simulink model "simulinkQ1b (1)"  (R2022a)
settings: Solver=VariableStepAuto  StartTime=0.0  StopTime=10.0  RelTol=1e-3
settings Model: Creator=ABHIJIT NIT  LastModifiedBy=heera
settings DebuggingCC: UnconnectedInputMsg=warning  UnconnectedOutputMsg=warning  UnconnectedLineMsg=warning
settings RTWCC: DLArmComputeVersion=19.05

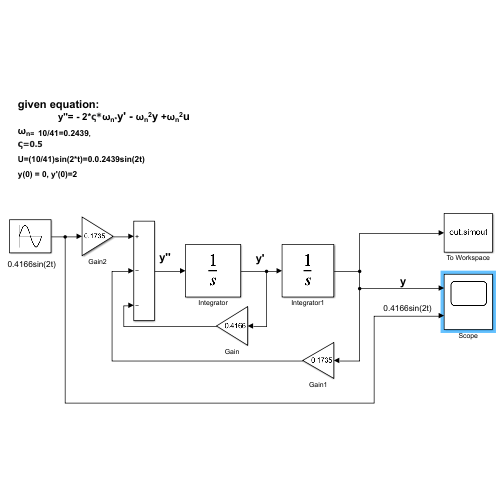
[thumbnail: Simulink's stored preview of the top-level diagram]
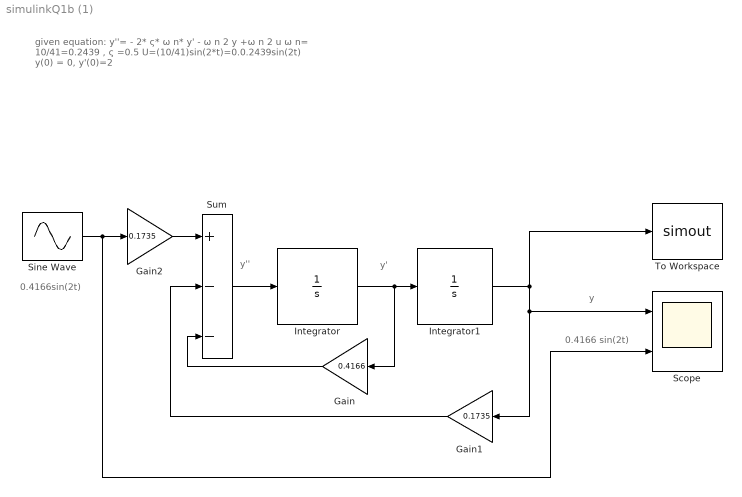
== system simulinkQ1b (1) ==
  note: 0.4166 sin(2t)
  note: 0.4166sin(2t)
  note: y''
  note: given equation:
      | y''= - 2* ς* ω n* y' - ω n 2 y +ω n 2 u
      | ω n= 10/41=0.2439 ,
      | ς =0.5
      | U=(10/41)sin(2*t)=0.0.2439sin(2t)
      | y(0) = 0, y'(0)=2
  note: y'
  note: y
  Gain : Gain  Gain=0.4166
  Gain1 : Gain  Gain=0.1735
  Gain2 : Gain  Gain=0.1735
  Integrator : Integrator  InitialCondition=2
  Integrator1 : Integrator
  Scope : Scope  NumInputPorts=2
  Sine Wave : Sin  Amplitude=0.4166  Frequency=2  SampleTime=0
  Sum : Sum  Inputs=+--
  To Workspace : ToWorkspace  VariableName=simout  SaveFormat=Timeseries  SampleTime=-1
  wires:
  Sum/1 -> Integrator/1
  Integrator/1 -> Integrator1/1, Gain/1
  Gain/1 -> Sum/3
  Integrator1/1 -> Scope/1, Gain1/1, To Workspace/1
  Gain1/1 -> Sum/2
  Sine Wave/1 -> Scope/2, Gain2/1
  Gain2/1 -> Sum/1
